simulink model "model_dynamic_feedback"  (R2023b)
settings: Solver=VariableStepAuto  StartTime=0.0  StopTime=10.0  RelTol=1e-3
libraries: simulink_extras x6, spspowerguiLib x1
settings Model: Creator=dimia  LastModifiedBy=dimia

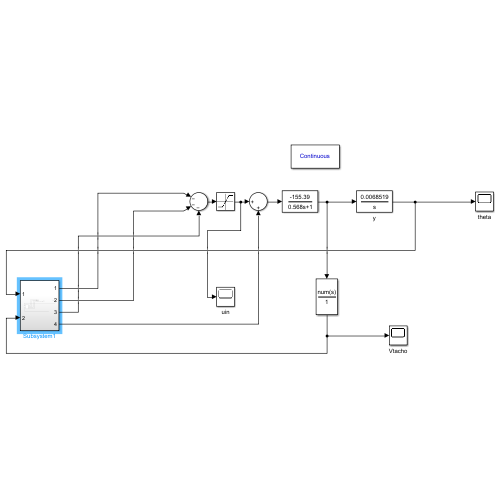
[thumbnail: Simulink's stored preview of the top-level diagram]
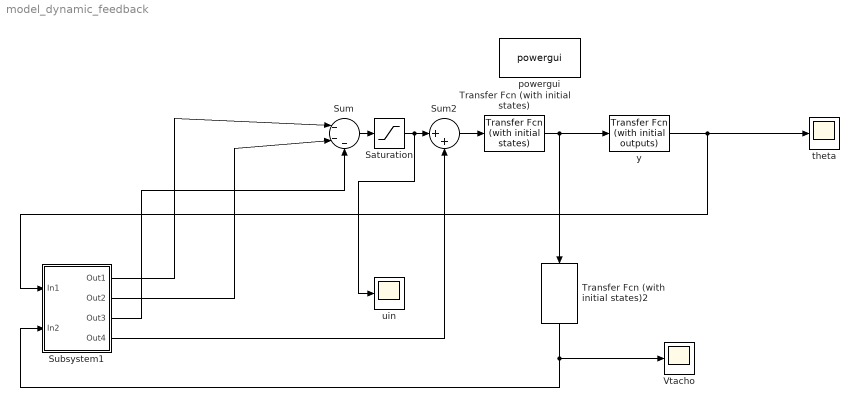
== system model_dynamic_feedback ==
  Saturation : Saturate  UpperLimit=10  LowerLimit=-10
  Subsystem1 : Subsystem
  Sum : Sum  Inputs=|---
  Sum2 : Sum  Inputs=|++
  Transfer Fcn (with initial states) : simulink_extras/Additional Linear/Transfer Fcn (with initial states)  N=[-155.39]  D="[0.568  1]"  X0=0
  Transfer Fcn (with initial states)2 : simulink_extras/Additional Linear/Transfer Fcn (with initial states)  N=-0.0001*9.2667  D=1  X0=0
  Vtacho : Scope
  powergui : spspowerguiLib/powergui  Priority=1  SimulationMode=Continuous  SampleTime=50e-6  frequency=60  Iterations=50  frequencyindice=60  Pbase=100e6  ErrMax=1e-4  UnitsV=kV  UnitsW=MW  buscounter=0  FunctionMessages=off  echomessages=off  EnableUseOfTLC=off  CurrentSourceSwitches=off  DisableSnubberDevices=off  DisableRonSwitches=off  DisableVfSwitches=off  DisplayEquations=off  AutomaticDiscreteSolvers=off  SolverType=Tustin/Backward Euler (TBE)  Interpol=off  ExternalGateDelay=off  methode=off  Ts=100  x0status=blocks  SPID=on  SwTol=0  HookPort=off  NonlinearTolerance=1e-4  nMaxIteration=100  ContinueOnMaxIteration=off  RestoreLinks=warning  ResistiveCurrentMeasurement=off  Frange=[0:2:500]  Ylog=off  Xlog=on  ShowGrid=off  save=off  variable=ZData  structure=0  ZoomFFT=off  StartTime=0.0  cycles=1  DisplayStyle=1  fundamental=60  FreqAxis=off  MaxFrequency=1000  frequencyindicesteady=1  RmsSteady=1  display=off
  theta : Scope
  uin : Scope
  y : simulink_extras/Additional Linear/Transfer Fcn (with initial outputs)  N=[(1/36)*0.24667]  D="[1  0]"  Y0=2  U0=0
  wires:
  y/1 -> Subsystem1/1(In1), theta/1
  Transfer Fcn (with initial states)/1 -> Transfer Fcn (with initial states)2/1, y/1
  Transfer Fcn (with initial states)2/1 -> Subsystem1/2(In2), Vtacho/1
  Sum2/1 -> Transfer Fcn (with initial states)/1
  Sum/1 -> Saturation/1
  Saturation/1 -> uin/1, Sum2/1
  Subsystem1/1(Out1) -> Sum/1
  Subsystem1/2(Out2) -> Sum/2
  Subsystem1/3(Out3) -> Sum/3
  Subsystem1/4(Out4) -> Sum2/2

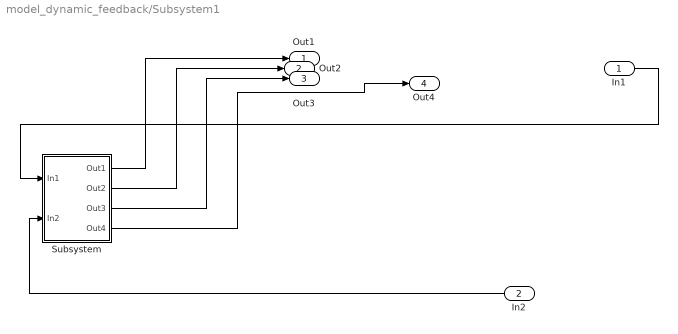
== system model_dynamic_feedback/Subsystem1 ==
  In1 : Inport
  In2 : Inport  Port=2
  Subsystem : Subsystem
  Out1 : Outport
  Out2 : Outport  Port=2
  Out3 : Outport  Port=3
  Out4 : Outport  Port=4
  wires:
  Subsystem/3(Out3) -> Out3/1
  Subsystem/2(Out2) -> Out2/1
  Subsystem/1(Out1) -> Out1/1
  In2/1 -> Subsystem/2(In2)
  In1/1 -> Subsystem/1(In1)
  Subsystem/4(Out4) -> Out4/1

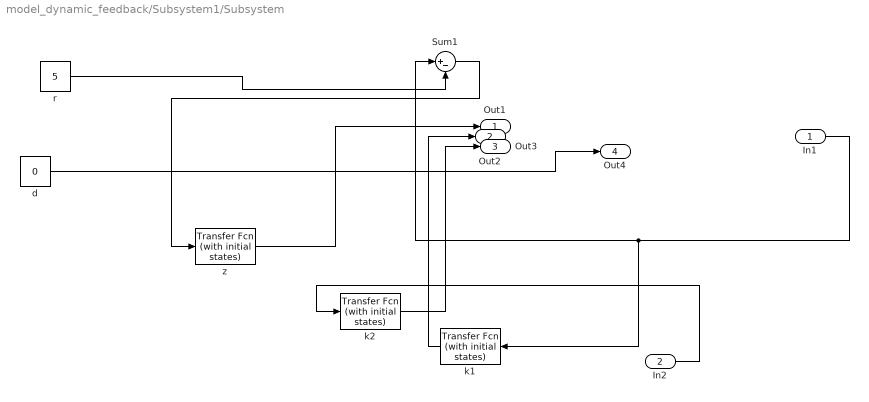
== system model_dynamic_feedback/Subsystem1/Subsystem ==
  In1 : Inport
  In2 : Inport  Port=2
  Sum1 : Sum  Inputs=|+-
  d : Constant  Value=0
  k1 : simulink_extras/Additional Linear/Transfer Fcn (with initial states)  N=[-14]  D=[1]  X0=0
  k2 : simulink_extras/Additional Linear/Transfer Fcn (with initial states)  N=[28]  D=[1]  X0=0
  r : Constant  Value=5
  z : simulink_extras/Additional Linear/Transfer Fcn (with initial states)  N=-14  D=[1 0]  X0=0
  Out1 : Outport
  Out2 : Outport  Port=2
  Out3 : Outport  Port=3
  Out4 : Outport  Port=4
  wires:
  r/1 -> Sum1/2
  In1/1 -> Sum1/1, k1/1
  Sum1/1 -> z/1
  k1/1 -> Out2/1
  k2/1 -> Out3/1
  In2/1 -> k2/1
  z/1 -> Out1/1
  d/1 -> Out4/1
